simulink subsystem "Bearing_Setup"  (R2021b)
settings: Solver=VariableStepAuto  StartTime=0.0  StopTime=10.0  RelTol=1e-3
settings Model: DefaultTestHarness=Bearing_Setup_Validation1  Creator=PhilippSchildt  LastModifiedBy=PhilippSchildt
settings SolverCC: AlgebraicLoopSolver=TrustRegion
settings DebuggingCC: SFMachineParentedDataDiag=warning

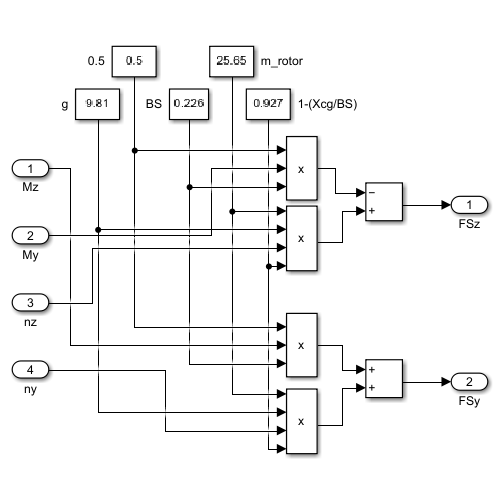
[thumbnail: Simulink's stored preview of the top-level diagram]
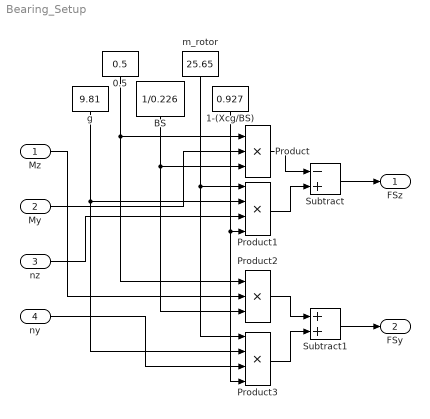
== system Bearing_Setup ==
  Mz : Inport
  My : Inport  Port=2
  nz : Inport  Port=3
  ny : Inport  Port=4
  0.5 : Constant  Value=0.5
  1-(Xcg/BS) : Constant  Value=0.927
  BS : Constant  Value=1/0.226
  Product : Product  Inputs=3
  Product1 : Product  Inputs=4
  Product2 : Product  Inputs=3
  Product3 : Product  Inputs=4
  Subtract : Sum  Inputs=-+
  Subtract1 : Sum
  g : Constant  Value=9.81
  m_rotor : Constant  Value=25.65
  FSz : Outport
  FSy : Outport  Port=2
  wires:
  Subtract/1 -> FSz/1
  Subtract1/1 -> FSy/1
  Product/1 -> Subtract/1
  Product1/1 -> Subtract/2
  0.5/1 -> Product2/1, Product/1
  Product3/1 -> Subtract1/2
  Product2/1 -> Subtract1/1
  My/1 -> Product/2
  BS/1 -> Product2/3, Product/3
  m_rotor/1 -> Product3/1, Product1/1
  g/1 -> Product1/2, Product3/2
  nz/1 -> Product1/3
  1-(Xcg/BS)/1 -> Product1/4, Product3/4
  Mz/1 -> Product2/2
  ny/1 -> Product3/3
